simulink model "DCMG2"  (R2014b)
settings: Solver=ode1  SolverMode=SingleTasking  StartTime=0.0  StopTime=Inf  FixedStep=Tm  RelTol=1e-3
PostLoadFcn:
  | , if any(exist('dsrtsu_mdlpostloadfcn', 'file') == [2, 3, 6]), try dsrtsu_mdlpostloadfcn('Execute', bdroot); catch fprintf('Error in PostLoadFcn (dsrtsu_mdlpostloadfcn) for model "%s":\n %s\n', bdroot, lasterr); end, end,
values from neighbouring files (symbols this model uses):
  C = 2200e-6    (= 0.0022)    [params.m]
  duty_boost = 250    [params.m]
  duty_hb = 1    [params.m]
  fixed_gain_ia = 10*(1/10e-3)    (= 1000)    [params.m]
  fixed_gain_ic = 10*(1/10e-3)    (= 1000)    [params.m]
  fixed_gain_vc1 = 10*200    (= 2000)    [params.m]
  fixed_gain_vc2 = 10*200    (= 2000)    [params.m]
  gain_ia = 1    [params.m]
  gain_ic = 1    [params.m]
  gain_vc1 = 1    [params.m]
  gain_vc2 = 1    [params.m]
  L = 12e-3    (= 0.012)    [params.m]
  offset_ia = 0    [params.m]
  offset_ic = 0    [params.m]
  offset_vc1 = -1.85    [params.m]
  offset_vc2 = 2.12    [params.m]
  R = 10    [params.m]
  S = [ ... (first row only)    [params.m]
  Tm = 30e-6    (= 3e-05)    [params.m]
libraries: rtilib1103 x9, simulink x4, rtitasklib x1
settings Model: DSRTSU_INTERNAL_RTI_VER=470  DSRTSU_INTERNAL_RTI_TYPE=rti1103  DSRTSU_INTERNAL_RTIFPGA=60  ExtModeTrigMode=oneshot  ExtModeArmWhenConnect=off  BufferReuse=off  Creator=USM  LastModifiedBy=Admin
settings DataIOCC: SignalLoggingSaveFormat=ModelDataLogs
settings OptimizationCC: BlockReduction=off  ConditionallyExecuteInputs=off  OptimizeBlockIOStorage=off  BufferReuse=off  GlobalBufferReuse=off  ExpressionFolding=off  ExpressionDepthLimit=2147483647  LocalBlockOutputs=off  InitFltsAndDblsToZero=on
settings DebuggingCC: SaveWithParameterizedLinksMsg=none  UnderspecifiedInitializationDetection=Classic  MergeDetectMultiDrivingBlocksExec=none  SignalResolutionControl=TryResolveAllWithWarning  MultiTaskDSMMsg=warning  MultiTaskCondExecSysMsg=none  MultiTaskRateTransMsg=warning  TasksWithSamePriorityMsg=none  FcnCallInpInsideContextMsg=UseLocalSettings  StateNameClashWarn=warning
settings HardwareCC: ProdLargestAtomicInteger=Integer  ProdLargestAtomicFloat=Float  ProdIntDivRoundTo=Zero  ProdEndianess=BigEndian  ProdHWDeviceType=Generic->Custom  TargetIntDivRoundTo=Zero  TargetEndianess=BigEndian  TargetHWDeviceType=Generic->Custom
settings RTWCC: SystemTargetFile=rti1103.tlc  MakeCommand=make_rti  TemplateMakefile=rti1103.tmf  Description=dSPACE DS1103 Hardware Platform  RTWVerbose=off  ProcessScript=rti1103_make_rtw_hook  IncludeERTFirstTime=on
settings STFCustomTargetCC: TargetFcnLib=ansi_tfl_tmw.mat  ParMdlRefBuildCompliant=on  GeneratePreprocessorConditionals=Disable all  CPPClassGenCompliant=on  SystemTargetFile=rti1103.tlc
settings GRTTargetCC: TargetFcnLib=ansi_tfl_tmw.mat  CompOptLevelCompliant=off  ConcurrentExecutionCompliant=off  CombineOutputUpdateFcns=off  MatFileLogging=off  GRTInterface=on  ExtModeMexFile=noextcomm

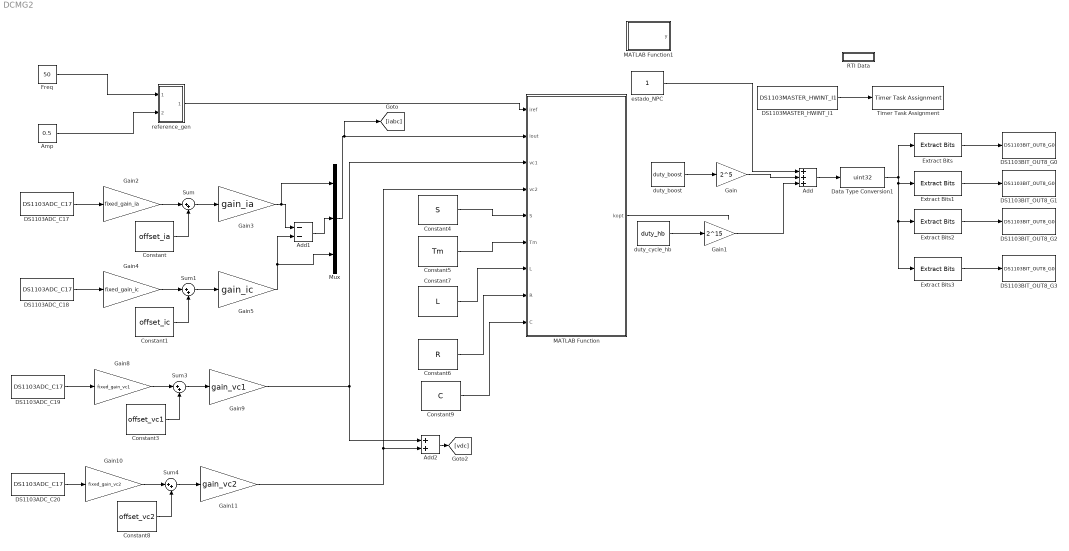
== system DCMG2 ==
  Add : Sum  Inputs=+++
  "Add1 " : Sum  Inputs=--
  Add2 : Sum
  Amp : Constant  Value=0.5
  Constant : Constant  Value=offset_ia
  Constant1 : Constant  Value=offset_ic
  Constant3 : Constant  Value=offset_vc1
  Constant4 : Constant  Value=S
  Constant5 : Constant  Value=Tm
  Constant6 : Constant  Value=R
  Constant7 : Constant  Value=L
  Constant8 : Constant  Value=offset_vc2
  Constant9 : Constant  Value=C
  DS1103ADC_C17 : rtilib1103/DS1103 MASTER PPC/DS1103ADC_C17  ChannelNo=17  TimerAPreTrigger=0  Reserved2=[]  Reserved3=[]  Reserved4=[]  DialogFcn=gui1103adc  UnitName={ 'DS1103ADC_C' }  UnitValues={ 17 }  DSProperties=struct('RTI',struct('Version',uint32(1),'BlockType',struct('isSLSource',uint8(1),'isSLSink',uint8(0),'isHWSource',uint8(1),'isHWSink',uint8(0),'isSetup',uint8(0),'isInline',uint8(1),'isNonInline',uint8(0),'isInterrupt',uint8(0),'isChannelwise',uint8(1)),'IOBoardType','DS1103MASTER','UnitType','ADC','Identifier','ADC','DialogType','ML','BlockSet','NONE','SlaveProcessor','NONE'))
  DS1103ADC_C18 : rtilib1103/DS1103 MASTER PPC/DS1103ADC_C17  ChannelNo=18  TimerAPreTrigger=0  Reserved2=[]  Reserved3=[]  Reserved4=[]  DialogFcn=gui1103adc  UnitName={ 'DS1103ADC_C' }  UnitValues={ 18 }  DSProperties=struct('RTI',struct('Version',uint32(1),'BlockType',struct('isSLSource',uint8(1),'isSLSink',uint8(0),'isHWSource',uint8(1),'isHWSink',uint8(0),'isSetup',uint8(0),'isInline',uint8(1),'isNonInline',uint8(0),'isInterrupt',uint8(0),'isChannelwise',uint8(1)),'IOBoardType','DS1103MASTER','UnitType','ADC','Identifier','ADC','DialogType','ML','BlockSet','NONE','SlaveProcessor','NONE'))
  DS1103ADC_C19 : rtilib1103/DS1103 MASTER PPC/DS1103ADC_C17  ChannelNo=19  TimerAPreTrigger=0  Reserved2=[]  Reserved3=[]  Reserved4=[]  DialogFcn=gui1103adc  UnitName={ 'DS1103ADC_C' }  UnitValues={ 19 }  DSProperties=struct('RTI',struct('Version',uint32(1),'BlockType',struct('isSLSource',uint8(1),'isSLSink',uint8(0),'isHWSource',uint8(1),'isHWSink',uint8(0),'isSetup',uint8(0),'isInline',uint8(1),'isNonInline',uint8(0),'isInterrupt',uint8(0),'isChannelwise',uint8(1)),'IOBoardType','DS1103MASTER','UnitType','ADC','Identifier','ADC','DialogType','ML','BlockSet','NONE','SlaveProcessor','NONE'))
  DS1103ADC_C20 : rtilib1103/DS1103 MASTER PPC/DS1103ADC_C17  ChannelNo=20  TimerAPreTrigger=0  Reserved2=[]  Reserved3=[]  Reserved4=[]  DialogFcn=gui1103adc  UnitName={ 'DS1103ADC_C' }  UnitValues={ 20 }  DSProperties=struct('RTI',struct('Version',uint32(1),'BlockType',struct('isSLSource',uint8(1),'isSLSink',uint8(0),'isHWSource',uint8(1),'isHWSink',uint8(0),'isSetup',uint8(0),'isInline',uint8(1),'isNonInline',uint8(0),'isInterrupt',uint8(0),'isChannelwise',uint8(1)),'IOBoardType','DS1103MASTER','UnitType','ADC','Identifier','ADC','DialogType','ML','BlockSet','NONE','SlaveProcessor','NONE'))
  DS1103BIT_OUT8_G0 : rtilib1103/DS1103 MASTER PPC/DS1103BIT_OUT8_G0  GroupNo=0  InitValue=0  TermMode=1  TermValue=0  Reserved1=[]  Reserved2=[]  Reserved3=[]  Reserved4=[]  DialogFcn=gui1103bit_out8  UnitName={ 'DS1103BIT_OUT8_G' }  UnitValues={ 0 }  DSProperties=struct('RTI',struct('Version',uint32(1),'BlockType',struct('isSLSource',uint8(0),'isSLSink',uint8(1),'isHWSource',uint8(0),'isHWSink',uint8(1),'isSetup',uint8(0),'isInline',uint8(1),'isNonInline',uint8(0),'isInterrupt',uint8(0),'isChannelwise',uint8(0)),'IOBoardType','DS1103MASTER','UnitType','BIT','Identifier','BITOUT8','DialogType','ML','BlockSet','NONE','SlaveProcessor','NONE'))
  DS1103BIT_OUT8_G1 : rtilib1103/DS1103 MASTER PPC/DS1103BIT_OUT8_G0  GroupNo=1  InitValue=0  TermMode=1  TermValue=0  Reserved1=[]  Reserved2=[]  Reserved3=[]  Reserved4=[]  DialogFcn=gui1103bit_out8  UnitName={ 'DS1103BIT_OUT8_G' }  UnitValues={1}  DSProperties=struct('RTI',struct('Version',uint32(1),'BlockType',struct('isSLSource',uint8(0),'isSLSink',uint8(1),'isHWSource',uint8(0),'isHWSink',uint8(1),'isSetup',uint8(0),'isInline',uint8(1),'isNonInline',uint8(0),'isInterrupt',uint8(0),'isChannelwise',uint8(0)),'IOBoardType','DS1103MASTER','UnitType','BIT','Identifier','BITOUT8','DialogType','ML','BlockSet','NONE','SlaveProcessor','NONE'))
  DS1103BIT_OUT8_G2 : rtilib1103/DS1103 MASTER PPC/DS1103BIT_OUT8_G0  GroupNo=2  InitValue=0  TermMode=1  TermValue=0  Reserved1=[]  Reserved2=[]  Reserved3=[]  Reserved4=[]  DialogFcn=gui1103bit_out8  UnitName={ 'DS1103BIT_OUT8_G' }  UnitValues={2}  DSProperties=struct('RTI',struct('Version',uint32(1),'BlockType',struct('isSLSource',uint8(0),'isSLSink',uint8(1),'isHWSource',uint8(0),'isHWSink',uint8(1),'isSetup',uint8(0),'isInline',uint8(1),'isNonInline',uint8(0),'isInterrupt',uint8(0),'isChannelwise',uint8(0)),'IOBoardType','DS1103MASTER','UnitType','BIT','Identifier','BITOUT8','DialogType','ML','BlockSet','NONE','SlaveProcessor','NONE'))
  DS1103BIT_OUT8_G3 : rtilib1103/DS1103 MASTER PPC/DS1103BIT_OUT8_G0  GroupNo=3  InitValue=0  TermMode=1  TermValue=0  Reserved1=[]  Reserved2=[]  Reserved3=[]  Reserved4=[]  DialogFcn=gui1103bit_out8  UnitName={ 'DS1103BIT_OUT8_G' }  UnitValues={3}  DSProperties=struct('RTI',struct('Version',uint32(1),'BlockType',struct('isSLSource',uint8(0),'isSLSink',uint8(1),'isHWSource',uint8(0),'isHWSink',uint8(1),'isSetup',uint8(0),'isInline',uint8(1),'isNonInline',uint8(0),'isInterrupt',uint8(0),'isChannelwise',uint8(0)),'IOBoardType','DS1103MASTER','UnitType','BIT','Identifier','BITOUT8','DialogType','ML','BlockSet','NONE','SlaveProcessor','NONE'))
  DS1103MASTER_HWINT_I1 : rtilib1103/DS1103 MASTER PPC/DS1103MASTER_HWINT_I1  Parameters=[]  TDef=[]  BoardType=[]  BoardIntNo=[]  InterruptName=[]  DisplayIntNo=[]  DialogFcn=[]  Reserved1=[]  Reserved2=[]  Reserved3=[]  Reserved4=[]  Revision=[]  UnitName=[]  UnitValues=[]  DSProperties=struct('RTI',struct('IOBoardType',{{'DS1103MASTER'}},'SlaveProcessor','NONE','UnitType','HWINT','Identifier','HWINT','Version',uint32(2),'BlockType',struct('isSLSource',uint8(1),'isSLSink',uint8(0),'isHWSource',uint8(1),'isHWSink',uint8(0),'isSetup',uint8(0),'isInline',uint8(1),'isNonInline',uint8(0),'isInterrupt',uint8(1),'isChannelwise',uint8(0)),'DialogType','ML','BlockSet','NONE','RelationId',struct('TH',struct('BlockId','HWINT'))))  RTIBlockInterface=struct('BlockName',struct('Token',{{'DS1103MASTER_HWINT_I'}},'BlockParam',{{'ThIntNo'}}),'BlockDisplay',{{['DS1103MASTER Board \nUser-Interrupt 1'],'center'}},'DialogFcn','rti110xhwintgui','OutputPortsActive',1,'OutputPortsWidth',int32(1),'FunctionCall',uint32(0),'OutputPortsName',{{[' ']}},'IconTransparency','on','InitLevel',3,'Options',{{'SS_OPTION_FORCE_NONINLINED_FCNCALL','SS_OPTION_ASYNCHRONOUS_INTERRUPT'}})  RTIBlockParameters=struct('BoardNo',{{0,'OFF',[]}},'ThIntNo',{{1,'ON',[1 13]}},'ThSrcSgnName',{{['User-Interrupt 1'],'OFF',[]}},'ThBlk',{{['struct(''blkh'',''DCMG2/DS1103MASTER_HWINT_I1'',''srcId'',''EXT0'',''srcSgnId'',''EXT0'',''intervalTmrBlockId'',[],''srcSgnName'',[''User-Interrupt 1''],''srcCpuId'','''',''isSrcCpu'',1,''isTargetCpu'',1,''srcOnMasterCpu'',1,''boardType'','''',''boardTypeNo'','''',''boardNo'',1,''intNo'',0,''subIntNo'',-1,''period'',0,''entryPoint'',''rti_EXT0'',''blockName'',''DS1103MASTER_HWINT_I1'',''taskNameDisplayExt'','''',''taskType'',''HWINT'',''groupId'',''HWINT'',''hookFcn'',''NULL'',''isTimerTaskSrc'',1,''service'','''',''mpBlkId'','''',''taskPriorityPreConfig'',''none'',''taskPriority'',-1,''taskSortWeighting'',[],''taskSchedulingPolicy'',''FCFS'',''taskOvrPreConfig'',''none'',''taskOvrStrategy'',1,''taskOvrQueueSize'',1,''taskVisibility'',''on'',''taskGroupId'','''',''taskGroupDisplayOrder'',[],''serviceDynamicGen'',0,''disableCodeGen'',0,''boardBase'',''0'',''noBoardBase'','''')'],'OFF',[]}},'TLCFileName',{{'rti_hwinterrupt','OFF',[]}},'PHSBoardBaseId',{{'DSXXXX','OFF',[]}})  RTISFcnParameters=struct('ThBlk','struct','ThIntNo','int32','TLCFileName','char','PHSBoardBaseId','char')  RTIBlockParaDefault=struct('BoardNo',0,'ThIntNo',1,'ThSrcSgnName',['User-Interrupt 1'],'ThBlk',['struct(''srcSgnId'', '''')'],'TLCFileName','rti_hwinterrupt','PHSBoardBaseId','DSXXXX')
  Data Type Conversion1 : DataTypeConversion  OutDataTypeStr=uint32
  Extract Bits : simulink/Logic and Bit Operations/Extract Bits  bitsToExtract=Range of bits  numBits=8  bitIdxRange=[0 7]  outScalingMode=Treat bit field as an integer
  Extract Bits1 : simulink/Logic and Bit Operations/Extract Bits  bitsToExtract=Range of bits  numBits=8  bitIdxRange=[8 15]  outScalingMode=Treat bit field as an integer
  Extract Bits2 : simulink/Logic and Bit Operations/Extract Bits  bitsToExtract=Range of bits  numBits=8  bitIdxRange=[16 23]  outScalingMode=Treat bit field as an integer
  Extract Bits3 : simulink/Logic and Bit Operations/Extract Bits  bitsToExtract=Range of bits  numBits=8  bitIdxRange=[24 31]  outScalingMode=Treat bit field as an integer
  Freq : Constant  Value=50
  Gain : Gain  Gain=2^5
  Gain1 : Gain  Gain=2^15
  Gain10 : Gain  Gain=fixed_gain_vc2
  Gain11 : Gain  Gain=gain_vc2
  Gain2 : Gain  Gain=fixed_gain_ia
  Gain3 : Gain  Gain=gain_ia
  Gain4 : Gain  Gain=fixed_gain_ic
  Gain5 : Gain  Gain=gain_ic
  Gain8 : Gain  Gain=fixed_gain_vc1
  Gain9 : Gain  Gain=gain_vc1
  MATLAB Function : MATLAB Function  TreatAsAtomicUnit=on
  MATLAB Function1 : MATLAB Function  TreatAsAtomicUnit=on
  Mux : Mux  Inputs=3
  RTI Data : Subsystem  Tag=struct('RTIDataServer',struct('RTIDataServerVs','2','RTIModelDescription','struct(''main'',''DCMG2'',''sub'','''',''isMp'',0)'))  LoadFcn="if exist('rtidc'), try,  rtidc('DataHostBlockClbLoad', gcbh); catch, disp(['Warning: ''LoadFcn'' for RTI Data block failed: ' lasterr]); end, end,"  mask(RTI_DATA_HOST){}
      mask help:
      | RTI Data Block.
      | This block is used by RTI to store internal model-dependent data.
      | Please keep this block on the root level of the model. Deleting this block will result in data loss.
      |
      | NEVER DELETE OR COPY THIS BLOCK!
      settings: CopyFcn="if exist('rtidc'), try,  rtidc('DataHostBlockClbCopy', gcbh); catch, disp(['Warning: ''CopyFcn'' for RTI Data block failed: ' lasterr]); end, end,"  DeleteFcn="if exist('rtidc'), try,  rtidc('DataHostBlockClbDelete', gcbh); catch, disp(['Warning: ''DeleteFcn'' for RTI Data block failed: ' lasterr]); end, end,"  ModelCloseFcn="if exist('rtidc'), try,  rtidc('DataHostBlockClbModelClose', gcbh); catch, disp(['Warning: ''ModelCloseFcn'' for RTI Data block failed: ' lasterr]); end, end,"  PreSaveFcn="if exist('rtidc'), try,  rtidc('DataHostBlockClbPreSave', gcbh); catch, disp(['Warning: ''PreSaveFcn'' for RTI Data block failed: ' lasterr]); end, end,"  PostSaveFcn="if exist('rtidc'), try,  rtidc('DataHostBlockClbPostSave', gcbh); catch, disp(['Warning: ''PostSaveFcn'' for RTI Data block failed: ' lasterr]); end, end,"  NameChangeFcn="if exist('rtidc'), try,  rtidc('DataHostBlockClbNameChange', gcbh); catch, disp(['Warning: ''NameChangeFcn'' for RTI Data block failed: ' lasterr]); end, end,"
      mask Help:
      | RTI Data Block.
      | This block is used by RTI to store internal model-dependent data.
      | Please keep this block on the root level of the model. Deleting this block will result in data loss.
      | 
      | NEVER DELETE OR COPY THIS BLOCK!
      mask Display:
      | text(0.5, 0.5, 'RTI Data', 'HorizontalAlignment', 'center');
      | plot([1 0]);
  Sum{,1,3..4} (4 alike) : Sum  Inputs=|++
  Timer Task Assignment : rtitasklib/Timer Task Assignment  Reserved2=[]  Reserved3=[]  Reserved4=[]  DSProperties=struct('RTI',struct('Version',uint32(2),'BlockType',struct('isSLSource',uint8(0),'isSLSink',uint8(1),'isHWSource',uint8(0),'isHWSink',uint8(0),'isSetup',uint8(0),'isInline',uint8(1),'isNonInline',uint8(0),'isInterrupt',uint8(0),'isChannelwise',uint8(0)),'IOBoardType','INTLIB','UnitType','TTASSIGN','Identifier','TTASSIGN','DialogType','SL','BlockSet','NONE','SlaveProcessor','NONE','RelationId',struct('TH',struct('BlockId','TTASSIGN'))))
  duty_boost : Constant  Value=duty_boost
  duty_cycle_hb : Constant  Value=duty_hb
  "estado_NPC " : Constant
  reference_gen : Subsystem
  wires:
  MATLAB Function/1(kopt) -> ?
  duty_cycle_hb/1 -> Gain1/1
  Gain/1 -> Add/2
  Gain1/1 -> Add/3
  Add/1 -> Data Type Conversion1/1
  Data Type Conversion1/1 -> Extract Bits/1, Extract Bits3/1, Extract Bits2/1, Extract Bits1/1
  Extract Bits/1 -> DS1103BIT_OUT8_G0/1
  Extract Bits1/1 -> DS1103BIT_OUT8_G1/1
  Extract Bits2/1 -> DS1103BIT_OUT8_G2/1
  Extract Bits3/1 -> DS1103BIT_OUT8_G3/1
  DS1103MASTER_HWINT_I1/1 -> Timer Task Assignment/1
  Freq/1 -> reference_gen/1(In1)
  Amp/1 -> reference_gen/2(In2)
  reference_gen/1(Out1) -> MATLAB Function/1(iref)
  DS1103ADC_C17/1 -> Gain2/1
  Gain2/1 -> Sum/1
  Constant/1 -> Sum/2
  Sum/1 -> Gain3/1
  DS1103ADC_C18/1 -> Gain4/1
  Gain4/1 -> Sum1/1
  Constant1/1 -> Sum1/2
  Sum1/1 -> Gain5/1
  Gain8/1 -> Sum3/1
  Constant3/1 -> Sum3/2
  Sum3/1 -> Gain9/1
  DS1103ADC_C19/1 -> Gain8/1
  Gain3/1 -> "Add1 "/1, Mux/1
  Gain5/1 -> Mux/3, "Add1 "/2
  Constant4/1 -> MATLAB Function/5(S)
  Constant5/1 -> MATLAB Function/6(Tm)
  Constant6/1 -> MATLAB Function/8(R)
  Constant7/1 -> MATLAB Function/7(L)
  Gain10/1 -> Sum4/1
  Constant8/1 -> Sum4/2
  Sum4/1 -> Gain11/1
  Gain11/1 -> Add2/2, MATLAB Function/4(vc2)
  DS1103ADC_C20/1 -> Gain10/1
  Constant9/1 -> MATLAB Function/9(C)
  Mux/1 -> [iabc], MATLAB Function/2(iout)
  Add2/1 -> [vdc]
  Gain9/1 -> Add2/1, MATLAB Function/3(vc1)
  duty_boost/1 -> Gain/1
  "Add1 "/1 -> Mux/2
  "estado_NPC "/1 -> Add/1

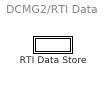
== system DCMG2/RTI Data ==
  RTI Data Store : Subsystem  Tag="struct('public',struct('sub',struct('name',{{'DCMG2'}},'data',{{struct('TH',struct('thTaskInfo',struct('taskType',{'TIMER','HWINT','TMRINT','SWINT','GLINT'},'tasksNumOf',{1,0,0,0,0},'srcIds',{{'EXT0'},{},{},{},{}},'taskNames',{{['Timer Task 1']},{},{},{},{}})),'th_tc',struct('dataType','TASK','taskGroupId','','taskGroupList',{{}},'taskSchedulingPolicy','FCFS','taskType','TIMER','blkh','DCMG2/DS1103MASTER_HWINT_I1','srcId','EXT0','srcSgnName',['User-Interrupt 1'],'srcCpuName','','taskName',['Timer Task 1  [3e-05] s'],'taskNameDisplayExt','','smplTime',3e-05,'smplTimeOffs',0,'hasFixedPriority',0,'priority',1,'hasFixedOvc',0,'ovcType',1,'ovcMax',1),'tc_th',struct('dataType','TASK','taskGroupId','','taskGroupList',{{}},'taskSchedulingPolicy','FCFS','taskType','TIMER','blkh','DCMG2/DS1103MASTER_HWINT_I1','srcId','EXT0','srcSgnName',['User-Interrupt 1'],'srcCpuName','','taskName',['Timer Task 1  [3e-05] s'],'taskNameDisplayExt','','smplTime',3e-05,'smplTimeOffs',0,'hasFixedPriority',0,'priority',1,'hasFixedOvc',0,'ovcType',1,'ovcMax',1))}})),'private',struct('version',struct('dsVer',uint32(2)),'access',struct('modified',['17-Oct-2024 12:46:06'],'type','Model','isPerm',1)))"  mask(RTI_DATA_STORE){}
      mask help:
      | RTI Data Store Block. This block is used by RTI to store internal model dependent data. Deleting this block will result in data loss.
      |
      | NEVER DELETE, COPY, OR MODIFY THIS BLOCK!
      mask Help:
      | RTI Data Store Block. This block is used by RTI to store internal model dependent data. Deleting this block will result in data loss.
      | 
      | NEVER DELETE, COPY, OR MODIFY THIS BLOCK!
      mask Display: text(0.5, 0.5, ' ', 'HorizontalAlignment', 'center');

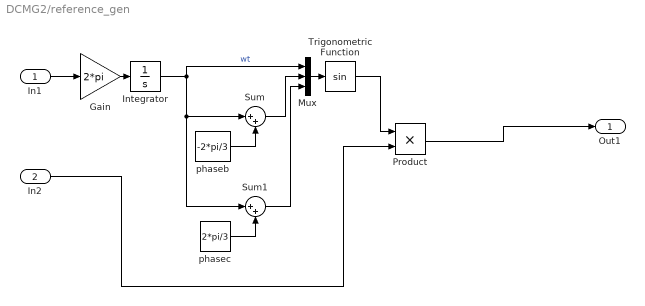
== system DCMG2/reference_gen ==
  In1 : Inport
  In2 : Inport  Port=2
  Gain : Gain  Gain=2*pi
  Integrator : Integrator
  Mux : Mux  Inputs=3
  Product : Product
  Sum : Sum  Inputs=|++
  Sum1 : Sum  Inputs=|++
  Trigonometric Function : Trigonometry
  phaseb : Constant  Value=-2*pi/3
  phasec : Constant  Value=2*pi/3
  Out1 : Outport
  wires:
  In1/1 -> Gain/1
  Sum/1 -> Mux/2
  Product/1 -> Out1/1
  Gain/1 -> Integrator/1
  In2/1 -> Product/2
  phaseb/1 -> Sum/2
  Trigonometric Function/1 -> Product/1
  phasec/1 -> Sum1/2
  Integrator/1 -> Sum1/1, Sum/1, Mux/1  "wt"
  Sum1/1 -> Mux/3
  Mux/1 -> Trigonometric Function/1

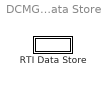
== system DCMG2/RTI Data/RTI Data Store ==
  RTI Data Store : Subsystem  mask(RTI_DATA_STORE){}
      mask help:
      | RTI Data Store Block. This block is used by RTI to store internal model dependent data. Deleting this block will result in data loss.
      |
      | NEVER DELETE, COPY, OR MODIFY THIS BLOCK!
      mask Help:
      | RTI Data Store Block. This block is used by RTI to store internal model dependent data. Deleting this block will result in data loss.
      | 
      | NEVER DELETE, COPY, OR MODIFY THIS BLOCK!
      mask Display: text(0.5, 0.5, ' ', 'HorizontalAlignment', 'center');

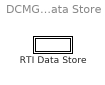
== system DCMG2/RTI Data/RTI Data Store/RTI Data Store ==
  RTI Data Store : Subsystem  mask(RTI_DATA_STORE){}
      mask help:
      | RTI Data Store Block. This block is used by RTI to store internal model dependent data. Deleting this block will result in data loss.
      |
      | NEVER DELETE, COPY, OR MODIFY THIS BLOCK!
      mask Help:
      | RTI Data Store Block. This block is used by RTI to store internal model dependent data. Deleting this block will result in data loss.
      | 
      | NEVER DELETE, COPY, OR MODIFY THIS BLOCK!
      mask Display: text(0.5, 0.5, ' ', 'HorizontalAlignment', 'center');

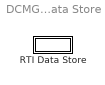
== system DCMG2/RTI Data/RTI Data Store/RTI Data Store/RTI Data Store ==
  RTI Data Store : Subsystem  mask(RTI_DATA_STORE){}
      mask help:
      | RTI Data Store Block. This block is used by RTI to store internal model dependent data. Deleting this block will result in data loss.
      |
      | NEVER DELETE, COPY, OR MODIFY THIS BLOCK!
      mask Help:
      | RTI Data Store Block. This block is used by RTI to store internal model dependent data. Deleting this block will result in data loss.
      | 
      | NEVER DELETE, COPY, OR MODIFY THIS BLOCK!
      mask Display: text(0.5, 0.5, ' ', 'HorizontalAlignment', 'center');

== system DCMG2/RTI Data/RTI Data Store/RTI Data Store/RTI Data Store/RTI Data Store ==

== matlab function DCMG2/MATLAB Function1 ==
  data: y output
function y = fcn()
persistent counter
if isempty(counter)
    counter = 1;
end

counter = counter + 1;
if(counter == 28)
    counter = 1;
end

y = counter;

== matlab function DCMG2/MATLAB Function ==
  data: iref input; iout input; vc1 input; vc2 input; kopt output; S input; Tm input; L input; R input; C input
function kopt  = fcn(iref, iout, vc1, vc2, S, Tm, L, R, C)
gmin = 100000000000;
kopt = 1;
for k = 1:27
    v = S(k,:)'*(vc1+vc2)/2;
    v = flip(v);
    vp = sum(v)/3;
    ikk = iout + (Tm/L)*(v-vp-R*iout);
    e = iref - ikk;

    if k<14
        if(all(S(k,:)<1))
            vkk2 = vc2*(1-Tm/(R*C));
            vkk1 = vc1 + vc2 - vkk2;
            ev = (vkk1-vkk2);
        else
            ev = vc1-vc2;
        end
    else
        if(all(S(k,:)>-1))
            vkk1 = vc1*(1-Tm/(R*C));
            vkk2 = vc1 + vc2 - vkk1;
            ev = (vkk1-vkk2);
        else
            ev = vc1-vc2;
        end
    end

    g = 100*ev*ev + e'*e;
    if g < gmin
        gmin = g;
        kopt = k;
    end
end
